simulink model "pendulum"  (R2025b)
settings: Solver=VariableStepAuto  StartTime=0.0  StopTime=100.0  FixedStep=0.02  RelTol=1e-3
settings Model: Creator=filip  LastModifiedBy=igorsiata
settings SolverCC: EnableFixedStepZeroCrossing=on

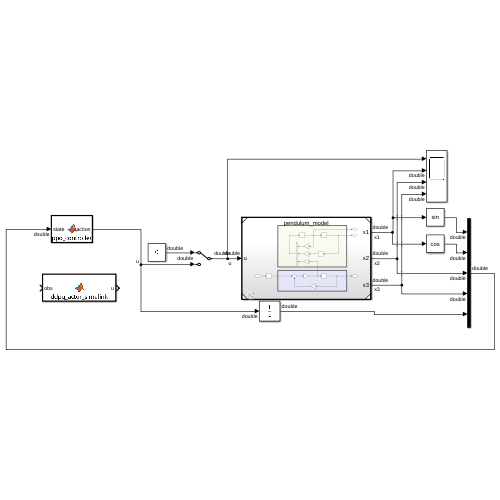
[thumbnail: Simulink's stored preview of the top-level diagram]
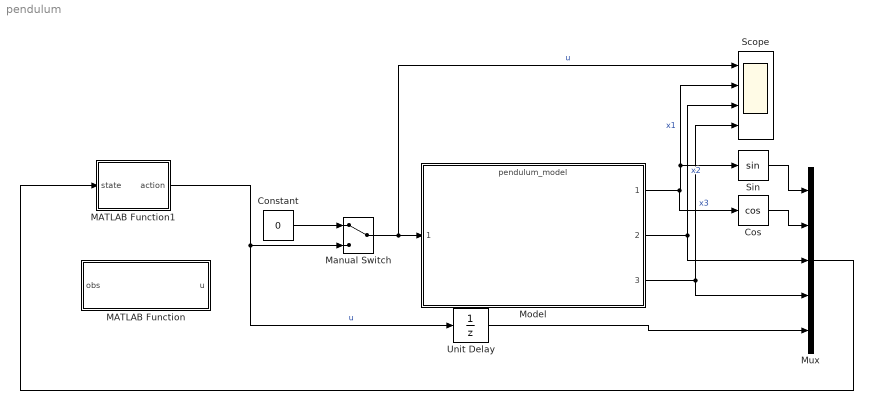
== system pendulum ==
  Constant : Constant  Value=0
  Cos : Trigonometry  Operator=cos
  MATLAB Function : MATLAB Function  TreatAsAtomicUnit=on
      settings: MinAlgLoopOccurrences=on
  MATLAB Function1 : MATLAB Function  TreatAsAtomicUnit=on
  Manual Switch : ManualSwitch
  Model : ModelReference  ModelNameDialog=pendulum_model.slx  SimulationMode=Normal  ModelReferenceVersion=1.6
  Mux : Mux  Inputs=5
  Scope : Scope  NumInputPorts=4
      settings: ActiveDisplayYMinimum=-1  ActiveDisplayYMaximum=1
  Sin : Trigonometry
  Unit Delay : UnitDelay  SampleTime=0.02  HasFrameUpgradeWarning=on
  wires:
  MATLAB Function1/1(action) -> Manual Switch/2, Unit Delay/1  "u"
  Model/2 -> Scope/3, Mux/3  "x2"
  Model/1 -> Cos/1, Sin/1, Scope/2  "x1"
  Model/3 -> Scope/4, Mux/4  "x3"
  Mux/1 -> MATLAB Function1/1(state)
  Unit Delay/1 -> Mux/5
  Constant/1 -> Manual Switch/1
  Manual Switch/1 -> Scope/1, Model/1  "u"
  Sin/1 -> Mux/1
  Cos/1 -> Mux/2

== matlab function pendulum/MATLAB Function ==
  data: obs input; u output
function u = ddpg_actor_simulink(obs)
u = 0;
% % DDPG Actor Network for Simulink
% % Input: obs = [theta; theta_dot; phi; prev_u] (4x1 column vector)
% % Output: u = applied action [-1, 1]
% % 
% % Must be called as MATLAB Function block with:
% %   - Input port: obs, [4, 1], double
% %   - Output port: u, scalar, double
% 
% persistent W1 b1 W2 b2 W3 b3 loaded
% 
% % Parameters
% du_max = 0.15;
% u_max = 1.0;
% 
% % Load weights on first call
% if isempty(loaded)
%         data = load('ddpg_actor_weights.mat');
%         W1 = double(data.layer0_weight);
%         b1 = double(data.layer0_bias(:));
%         W2 = double(data.layer1_weight);
%         b2 = double(data.layer1_bias(:));
%         W3 = double(data.layer2_weight);
%         b3 = double(data.layer2_bias(:));
%         loaded = true;
% end
% 
% % Extract observation components
% theta = obs(1);
% theta_dot = obs(2);
% phi = obs(3);
% prev_u = obs(4);
% 
% % Normalize angle to [-pi, pi]
% theta = wrap_angle(theta);
% 
% % Create input vector (column vector, 3x1)
% x = [theta; theta_dot; phi];
% 
% % Forward pass through network
% % Layer 1: 3 -> 400 with ReLU
% h1 = max(0, W1 * x + b1);  % [400, 3] * [3, 1] = [400, 1]
% 
% % Layer 2: 400 -> 300 with ReLU
% h2 = max(0, W2 * h1 + b2);  % [300, 400] * [400, 1] = [300, 1]
% 
% % Layer 3: 300 -> 1 with Tanh
% u_cmd = tanh(W3 * h2 + b3);  % [1, 300] * [300, 1] = [1, 1]
% 
% % Convert to scalar
% u_cmd = double(u_cmd);
% if isa(u_cmd, 'double') && numel(u_cmd) > 1
%     u_cmd = u_cmd(1);
% end
% 
% % Apply rate limiter (slew-rate limiting)
% u_low = prev_u - du_max;
% u_high = prev_u + du_max;
% u = min(max(u_cmd, u_low), u_high);
% 
% % Saturate to motor limits
% u = min(max(u, -u_max), u_max);
% 
% end
% 
% function y = wrap_angle(x)
% % Wrap angle to [-pi, pi)
% % Codegen-safe implementation for Simulink
% y = mod(x + pi, 2*pi) - pi;
end

== matlab function pendulum/MATLAB Function1 ==
  data: state input; action output
function action = ppo_controller(state)
    %#codegen
    
    % coder.load działa TYLKO przy generowaniu kodu (lub w symulacji). 
    % Zwraca strukturę z zawartością pliku .mat.
    % Kompilator zoptymalizuje to i wygeneruje statyczne tablice w kodzie C.
    weights = coder.load('ppo_actor_weights.mat');
    
    % Rzutowanie wejścia
    x = single(state); 
    
    z1 = weights.actor_net_0_weight * x + weights.actor_net_0_bias;
    a1 = tanh(z1); 
    z2 = weights.actor_net_2_weight * a1 + weights.actor_net_2_bias;
    a2 = tanh(z2); 
    z3 = weights.actor_net_4_weight * a2 + weights.actor_net_4_bias;

    action = double(z3);
end
